simulink model "Model_integrated"  (R2016b)
settings: Solver=VariableStepAuto  StartTime=0.0  StopTime=20  MaxStep=0.01  MinStep=.005  RelTol=1e-4  EnableMultiTasking=on
libraries: simulink x8
settings Model: Creator=Issac Ross  LastModifiedBy=Issac Ross
settings DataIOCC: SaveOutput=off  SaveTime=off
settings OptimizationCC: ExpressionDepthLimit=2147483647  LifeSpan=1
settings DebuggingCC: UnderspecifiedInitializationDetection=Classic  MergeDetectMultiDrivingBlocksExec=none  FcnCallInpInsideContextMsg=warning  AllowSymbolicDim=off  StateNameClashWarn=warning  SFUnexpectedBacktrackingDiag=warning  SFNoUnconditionalDefaultTransitionDiag=warning  SFExecutionAtInitializationDiag=none
settings GRTTargetCC: TargetLangStandard=C89/C90 (ANSI)  GeneratePreprocessorConditionals=Disable all  CombineOutputUpdateFcns=off  GRTInterface=on

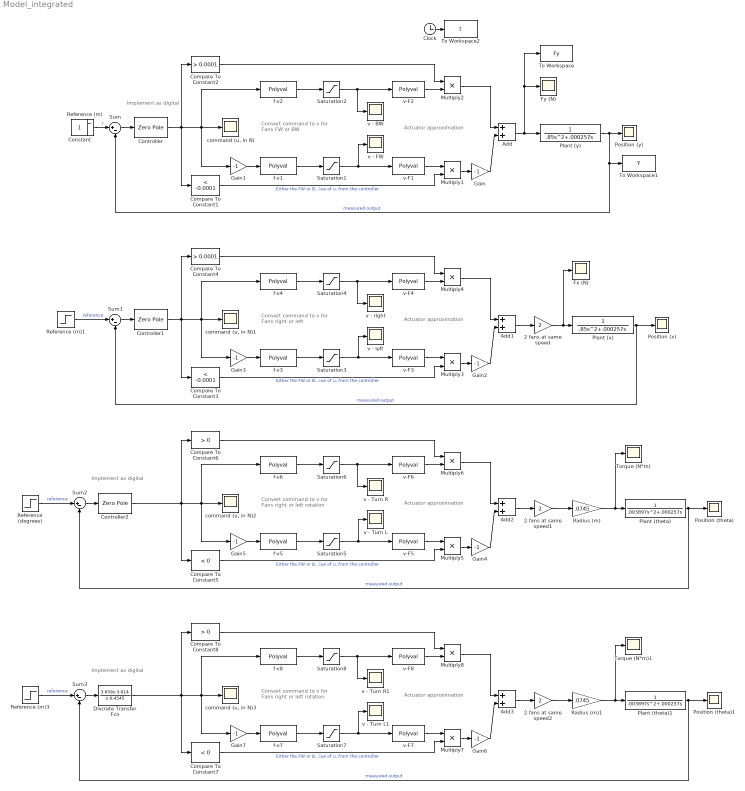
== system Model_integrated ==
  note: Implement as digital
  note: Actuator approximation
  note: Convert command to v
      | for Fans FW or BW
  note: Actuator approximation
  note: Convert command to v
      | for Fans right or left
  note: Implement as digital
  note: Actuator approximation
  note: Convert command to v
      | for Fans right or left rotation
  note: Implement as digital
  note: Actuator approximation
  note: Convert command to v
      | for Fans right or left rotation
  2 fans at same speed : Gain  Gain=2
  2 fans at same speed1 : Gain  Gain=2
  2 fans at same speed2 : Gain  Gain=2
  Add{,1..3} (4 alike) : Sum
  Clock : Clock
  Compare To Constant1 : simulink/Logic and Bit Operations/Compare To Constant  relop=<  const=-0.0001  OutDataTypeStr=uint8  ZeroCross=off
  Compare To Constant2 : simulink/Logic and Bit Operations/Compare To Constant  relop=>  const=0.0001  OutDataTypeStr=uint8  ZeroCross=off
  Compare To Constant3 : simulink/Logic and Bit Operations/Compare To Constant  relop=<  const=-0.0001  OutDataTypeStr=uint8  ZeroCross=off
  Compare To Constant4 : simulink/Logic and Bit Operations/Compare To Constant  relop=>  const=0.0001  OutDataTypeStr=uint8  ZeroCross=off
  Compare To Constant5 : simulink/Logic and Bit Operations/Compare To Constant  relop=<  const=0  OutDataTypeStr=uint8  ZeroCross=off
  Compare To Constant6 : simulink/Logic and Bit Operations/Compare To Constant  relop=>  const=0  OutDataTypeStr=uint8  ZeroCross=off
  Compare To Constant7 : simulink/Logic and Bit Operations/Compare To Constant  relop=<  const=0  OutDataTypeStr=uint8  ZeroCross=off
  Compare To Constant8 : simulink/Logic and Bit Operations/Compare To Constant  relop=>  const=0  OutDataTypeStr=uint8  ZeroCross=off
  Controller : ZeroPole  Zeros=[-.21]  Poles=[-10]  Gain=[6]
  Controller1 : ZeroPole  Zeros=[-.315]  Poles=[-5]  Gain=[3]
  Controller2 : ZeroPole  Zeros=[-.25]  Poles=[-15]  Gain=[.5]
  Discrete Transfer Fcn : DiscreteTransferFcn  Numerator=[3.659 -3.614]  Denominator=[1 -0.4545]  SampleTime=.05
  Fx (N) : Scope
  Fy (N) : Scope
  Gain{,1..7} (8 alike) : Gain  Gain=-1
  Multiply{1..8} (8 alike) : Product  Inputs=**
  Plant (theta) : TransferFcn  Denominator=[.003897 .000257 0]
  Plant (theta)1 : TransferFcn  Denominator=[.003897 .000257 0]
  Plant (x) : TransferFcn  Denominator=[.85 .000257 0]
  Plant (y) : TransferFcn  Denominator=[.85 .000257 0]
  Position (theta) : Scope
  Position (theta)1 : Scope
  Position (x) : Scope
  Position (y) : Scope
  Radius (m) : Gain  Gain=.0745
  Radius (m)1 : Gain  Gain=.0745
  Reference (degrees) : Step  Time=0  After=40  SampleTime=0
  Reference (m) : Step  Time=0  SampleTime=0
  Reference (m)1 : Step  Time=0  SampleTime=0
  Reference (m)3 : Step  Time=0  After=90  SampleTime=0
  Saturation{1..4} (4 alike) : Saturate  UpperLimit=255  LowerLimit=0  LinearizeAsGain=off  ZeroCross=off
  Saturation{5..8} (4 alike) : Saturate  UpperLimit=255  LowerLimit=50  LinearizeAsGain=off  ZeroCross=off
  Sum{,1..3} (4 alike) : Sum  Inputs=|+-
  To Workspace : ToWorkspace  VariableName=Fy  SampleTime=-1
  To Workspace1 : ToWorkspace  VariableName=Y  SampleTime=-1
  To Workspace2 : ToWorkspace  VariableName=t  SampleTime=-1
  Torque (N*m) : Scope
  Torque (N*m)1 : Scope
  command (u, in N){,1..3} (4 alike) : Scope
  f-v{1..8} (8 alike) : Polyval  Coefs=[1.66e004 49]
  v - BW : Scope
  v - FW : Scope
  v - Turn L : Scope
  v - Turn L1 : Scope
  v - Turn R : Scope
  v - Turn R1 : Scope
  v - left : Scope
  v - right : Scope
  v-F{1..8} (8 alike) : Polyval  Coefs=[5.63e-005 -2.29e-003]
  Constant : Constant  IOType=siggen
  wires:
  Reference (m)/1 -> Sum/1  "r"
  Plant (y)/1 -> Position (y)/1, To Workspace1/1, Sum/2  "measured output"
  Sum/1 -> Controller/1
  Gain1/1 -> f-v1/1
  Gain/1 -> Add/2
  Multiply1/1 -> Gain/1
  v-F1/1 -> Multiply1/1
  Compare To Constant1/1 -> Multiply1/2  "Either the FW or BW fan is necessary depending on value of u, from the controller"
  Multiply2/1 -> Add/1
  v-F2/1 -> Multiply2/2
  Compare To Constant2/1 -> Multiply2/1
  f-v2/1 -> Saturation2/1
  f-v1/1 -> Saturation1/1
  Saturation1/1 -> v-F1/1, v - FW/1
  Saturation2/1 -> v-F2/1, v - BW/1
  Add/1 -> Plant (y)/1, To Workspace/1, Fy (N)/1
  Controller/1 -> Compare To Constant2/1, Gain1/1, f-v2/1, "command (u, in N)"/1, Compare To Constant1/1
  Reference (m)1/1 -> Sum1/1  "reference"
  Plant (x)/1 -> Sum1/2, Position (x)/1  "measured output"
  Sum1/1 -> Controller1/1
  Gain3/1 -> f-v3/1
  Gain2/1 -> Add1/2
  Multiply3/1 -> Gain2/1
  v-F3/1 -> Multiply3/1
  Compare To Constant3/1 -> Multiply3/2  "Either the FW or BW fan is necessary depending on value of u, from the controller"
  Multiply4/1 -> Add1/1
  v-F4/1 -> Multiply4/2
  Compare To Constant4/1 -> Multiply4/1
  f-v4/1 -> Saturation4/1
  f-v3/1 -> Saturation3/1
  Saturation3/1 -> v-F3/1, v - left/1
  Saturation4/1 -> v-F4/1, v - right/1
  Add1/1 -> 2 fans at same speed/1
  Controller1/1 -> Compare To Constant4/1, Gain3/1, f-v4/1, "command (u, in N)1"/1, Compare To Constant3/1
  2 fans at same speed/1 -> Fx (N)/1, Plant (x)/1
  Reference (degrees)/1 -> Sum2/1  "reference"
  Plant (theta)/1 -> Sum2/2, Position (theta)/1  "measured output"
  Sum2/1 -> Controller2/1
  Gain5/1 -> f-v5/1
  Gain4/1 -> Add2/2
  Multiply5/1 -> Gain4/1
  v-F5/1 -> Multiply5/1
  Compare To Constant5/1 -> Multiply5/2  "Either the FW or BW fan is necessary depending on value of u, from the controller"
  Multiply6/1 -> Add2/1
  v-F6/1 -> Multiply6/2
  Compare To Constant6/1 -> Multiply6/1
  f-v6/1 -> Saturation6/1
  f-v5/1 -> Saturation5/1
  Saturation5/1 -> v-F5/1, v - Turn L/1
  Saturation6/1 -> v-F6/1, v - Turn R/1
  Add2/1 -> 2 fans at same speed1/1
  Controller2/1 -> Compare To Constant6/1, Gain5/1, f-v6/1, "command (u, in N)2"/1, Compare To Constant5/1
  2 fans at same speed1/1 -> Radius (m)/1
  Radius (m)/1 -> Torque (N*m)/1, Plant (theta)/1
  Reference (m)3/1 -> Sum3/1  "reference"
  Plant (theta)1/1 -> Sum3/2, Position (theta)1/1  "measured output"
  Sum3/1 -> Discrete Transfer Fcn/1
  Gain7/1 -> f-v7/1
  Gain6/1 -> Add3/2
  Multiply7/1 -> Gain6/1
  v-F7/1 -> Multiply7/1
  Compare To Constant7/1 -> Multiply7/2  "Either the FW or BW fan is necessary depending on value of u, from the controller"
  Multiply8/1 -> Add3/1
  v-F8/1 -> Multiply8/2
  Compare To Constant8/1 -> Multiply8/1
  f-v8/1 -> Saturation8/1
  f-v7/1 -> Saturation7/1
  Saturation7/1 -> v-F7/1, v - Turn L1/1
  Saturation8/1 -> v-F8/1, v - Turn R1/1
  Add3/1 -> 2 fans at same speed2/1
  Discrete Transfer Fcn/1 -> Compare To Constant8/1, Gain7/1, f-v8/1, "command (u, in N)3"/1, Compare To Constant7/1
  2 fans at same speed2/1 -> Radius (m)1/1
  Radius (m)1/1 -> Torque (N*m)1/1, Plant (theta)1/1
  Clock/1 -> To Workspace2/1
